simulink model "mass_spring_damper_simple"  (R2020a)
settings: Solver=VariableStepAuto  StartTime=0.0  StopTime=10.0  RelTol=1e-9
settings Model: Creator=USUARIO  LastModifiedBy=USUARIO

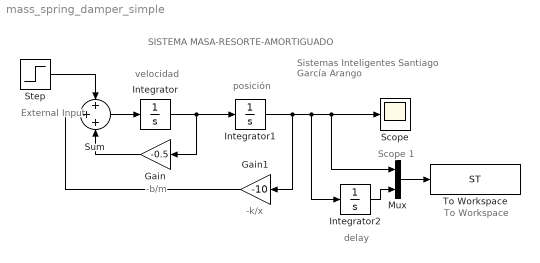
== system mass_spring_damper_simple ==
  note: Sistemas Inteligentes
      | Santiago García Arango
  note: SISTEMA MASA-RESORTE-AMORTIGUADO
  note: Scope 1
  note: To Workspace
  note: External
      | Input
  note: velocidad
  note: posición
  note: -b/m
  note: -k/x
  note: delay
  Gain : Gain  Gain=-0.5
  Gain1 : Gain  Gain=-10
  Integrator : Integrator
  Integrator1 : Integrator  InitialCondition=1
  Integrator2 : Integrator
  Mux : Mux  Inputs=2
  Scope : Scope
  Step : Step  Before=1  After=0  SampleTime=0
  Sum : Sum  Inputs=+++
  To Workspace : ToWorkspace  VariableName=ST  SampleTime=-1
  wires:
  Sum/1 -> Integrator/1
  Integrator/1 -> Integrator1/1, Gain/1
  Integrator1/1 -> Integrator2/1, Mux/1, Scope/1, Gain1/1
  Gain/1 -> Sum/3
  Gain1/1 -> Sum/2
  Step/1 -> Sum/1
  Mux/1 -> To Workspace/1
  Integrator2/1 -> Mux/2
